simulink model "EngineModel_student2"  (R2016a)
settings: Solver=ode3  StartTime=0.0  StopTime=1*sim_time  FixedStep=stepsize  RelTol=1e-3
values from neighbouring files (symbols this model uses):
  AFR_effective = max(AFR_stoich,AFR)    [EM3.m]    (also in workspace.mat = 14.7)
  Bore = 73.4*10^-3    (= 0.0734)    [EM3.m]    (also in workspace.mat)
  Cd = 0.35    [EM3.m]    (also in workspace.mat)
  ConRod = 137.2*10^-3    (= 0.1372)    [EM3.m]    (also in workspace.mat)
  CrankRadius = Stroke/2    (= 0.0363)    [EM3.m]    (also in workspace.mat)
  engine_speed = 3000    [EM3.m]    (also in workspace.mat)
  gma = 1.32    [EM3.m]    (also in workspace.mat)
  LHV = 44400*10^3    (= 44400000)    [EM3.m]    (also in workspace.mat)
  m_0 = P_0*(V_comp)/(R*T_air)    (= 3.64160478062e-05)    [EM3.m]    (also in workspace.mat)
  MAP = 80000    [EM3.m]    (also in workspace.mat)
  Nr_of_valves = 2    [EM3.m]    (also in workspace.mat)
  P_0 = 100000    [EM3.m]    (also in workspace.mat)
  P_exhaust = 120000    [EM3.m]    (also in workspace.mat)
  R = 287    [EM3.m]    (also in workspace.mat)
  Rho = 1.27    [EM3.m]    (also in workspace.mat)
  T_air = 323    [EM3.m]    (also in workspace.mat)
  V_comp = V_cyl/(CR-1)    (= 3.37580404769e-05)    [EM3.m]    (also in workspace.mat)
  V_sonic = 20.0457*sqrt(T_air)    [EM3.m]    (also in workspace.mat = 360.265344687)
  Valve_dia = 30*10^-3    (= 0.03)    [EM3.m]    (also in workspace.mat)
  Valve_lift = 9*10^-3    (= 0.009)    [EM3.m]    (also in workspace.mat)
settings Model: Creator=htsauto  LastModifiedBy=Job
settings DataIOCC: LimitDataPoints=on  SaveFormat=Array  SignalLoggingSaveFormat=ModelDataLogs
settings OptimizationCC: ExpressionDepthLimit=2147483647
settings DebuggingCC: UnderspecifiedInitializationDetection=Classic  MergeDetectMultiDrivingBlocksExec=none  SolverPrmCheckMsg=warning  FcnCallInpInsideContextMsg=UseLocalSettings  StateNameClashWarn=warning
settings HardwareCC: ProdBitPerPointer=32  ProdLargestAtomicFloat=None  ProdIntDivRoundTo=Undefined  ProdEndianess=Unspecified  ProdWordSize=32  ProdHWDeviceType=32-bit Generic
settings ModelReferenceCC: PropagateSignalLabelsOutOfModel=off
settings GRTTargetCC: CombineOutputUpdateFcns=off  GRTInterface=on
settings ConfigComp: CovModelRefEnable=Off  CovSFcnEnable=off

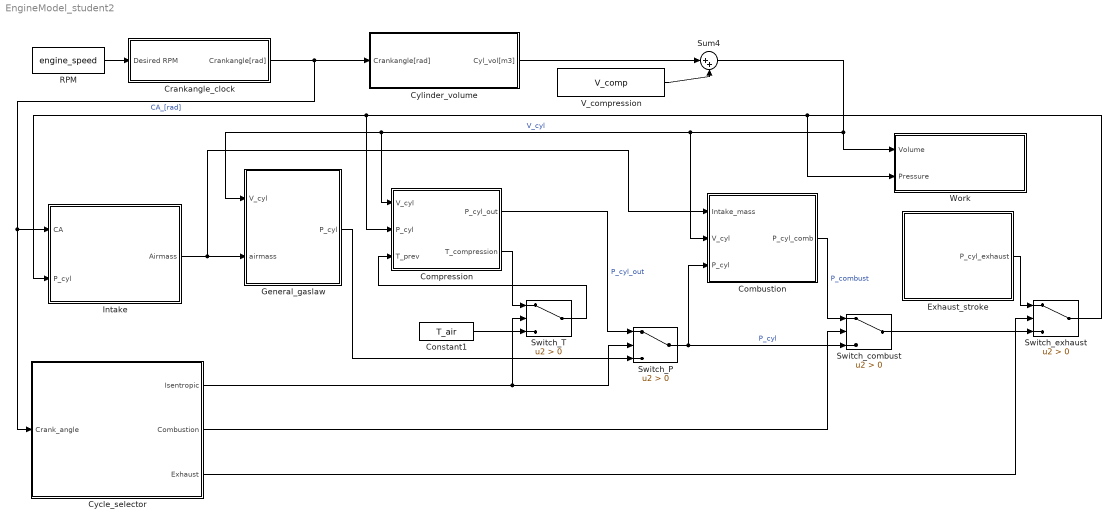
== system EngineModel_student2 ==
  Combustion : Subsystem
  Compression : Subsystem
  Constant1 : Constant  Value=T_air
  Crankangle_clock : Subsystem
  Cycle_selector : Subsystem
  Cylinder_volume : Subsystem
  Exhaust_stroke : Subsystem
  General_gaslaw : Subsystem
  Intake : Subsystem
  RPM : Constant  Value=engine_speed
  Sum4 : Sum  Inputs=|++
  Switch_P : Switch  Criteria=u2 > Threshold
  Switch_T : Switch  Criteria=u2 > Threshold
  Switch_combust : Switch  Criteria=u2 > Threshold
  Switch_exhaust : Switch  Criteria=u2 > Threshold
  V_compression : Constant  Value=V_comp
  Work : Subsystem
  wires:
  Sum4/1 -> Combustion/2(V_cyl), General_gaslaw/1(V_cyl), Compression/1(V_cyl), Work/1(Volume)  "V_cyl"
  RPM/1 -> Crankangle_clock/1(Desired RPM)
  Compression/1(P_cyl_out) -> Switch_P/1  "P_cyl_out"
  Compression/2(T_compression) -> Switch_T/1
  Switch_P/1 -> Switch_combust/3, Combustion/3(P_cyl)  "P_cyl"
  Combustion/1(P_cyl_comb) -> Switch_combust/1  "P_combust"
  Crankangle_clock/1(Crankangle[rad]) -> Cycle_selector/1(Crank_angle), Intake/1(CA), Cylinder_volume/1(Crankangle[rad])  "CA_[rad]"
  Switch_combust/1 -> Switch_exhaust/3
  Exhaust_stroke/1(P_cyl_exhaust) -> Switch_exhaust/1
  Cycle_selector/2(Combustion) -> Switch_combust/2
  Cycle_selector/3(Exhaust) -> Switch_exhaust/2
  Intake/1(Airmass) -> Combustion/1(Intake_mass), General_gaslaw/2(airmass)
  General_gaslaw/1(P_cyl) -> Switch_P/3
  Switch_exhaust/1 -> Work/2(Pressure), Intake/2(P_cyl), Compression/2(P_cyl)
  Switch_T/1 -> Compression/3(T_prev)
  Constant1/1 -> Switch_T/3
  Cycle_selector/1(Isentropic) -> Switch_P/2, Switch_T/2
  Cylinder_volume/1(Cyl_vol[m3]) -> Sum4/1
  V_compression/1 -> Sum4/2

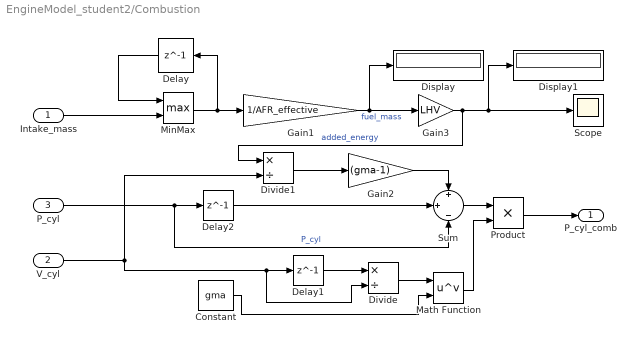
== system EngineModel_student2/Combustion ==
  Intake_mass : Inport
  V_cyl : Inport  Port=2
  P_cyl : Inport  Port=3
  Constant : Constant  Value=gma
  Delay : Delay  DelayLength=1  InitialCondition=0
  Delay1 : Delay  DelayLength=1
  Delay2 : Delay  DelayLength=1
  Display : Display
  Display1 : Display
  Divide : Product  Inputs=*/
  Divide1 : Product  Inputs=*/
  Gain1 : Gain  Gain=1/AFR_effective
  Gain2 : Gain  Gain=(gma-1)
  Gain3 : Gain  Gain=LHV
  Math Function : Math  Operator=pow  SaturateOnIntegerOverflow=on
  MinMax : MinMax  Function=max  Inputs=2
  Product : Product
  Scope : Scope
  Sum : Sum  Inputs=+|+|-
  P_cyl_comb : Outport
  wires:
  Intake_mass/1 -> MinMax/2
  MinMax/1 -> Delay/1, Gain1/1
  Gain1/1 -> Gain3/1, Display/1  "fuel_mass"
  Gain3/1 -> Scope/1, Display1/1, Divide1/1  "added_energy"
  Delay/1 -> MinMax/1
  Delay1/1 -> Divide/1
  Divide/1 -> Math Function/1
  Constant/1 -> Math Function/2
  Product/1 -> P_cyl_comb/1
  V_cyl/1 -> Divide1/2, Divide/2, Delay1/1
  P_cyl/1 -> Sum/3, Delay2/1  "P_cyl"
  Divide1/1 -> Gain2/1
  Sum/1 -> Product/1
  Gain2/1 -> Sum/1
  Delay2/1 -> Sum/2
  Math Function/1 -> Product/2

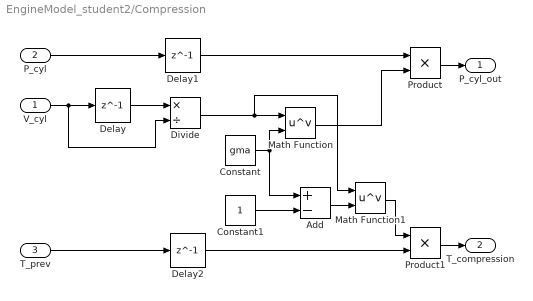
== system EngineModel_student2/Compression ==
  V_cyl : Inport
  P_cyl : Inport  Port=2
  T_prev : Inport  Port=3
  Add : Sum  Inputs=+-
  Constant : Constant  Value=gma
  Constant1 : Constant
  Delay : Delay  DelayLength=1  InitialCondition=0
  Delay1 : Delay  DelayLength=1
  Delay2 : Delay  DelayLength=1
  Divide : Product  Inputs=*/
  Math Function : Math  Operator=pow  SaturateOnIntegerOverflow=on
  Math Function1 : Math  Operator=pow  SaturateOnIntegerOverflow=on
  Product : Product
  Product1 : Product
  P_cyl_out : Outport
  T_compression : Outport  Port=2
  wires:
  V_cyl/1 -> Delay/1, Divide/2
  Math Function/1 -> Product/2
  Constant/1 -> Math Function/2, Add/1
  Constant1/1 -> Add/2
  Add/1 -> Math Function1/2
  Math Function1/1 -> Product1/1
  Product1/1 -> T_compression/1
  P_cyl/1 -> Delay1/1
  Divide/1 -> Math Function1/1, Math Function/1
  T_prev/1 -> Delay2/1
  Product/1 -> P_cyl_out/1
  Delay/1 -> Divide/1
  Delay1/1 -> Product/1
  Delay2/1 -> Product1/2

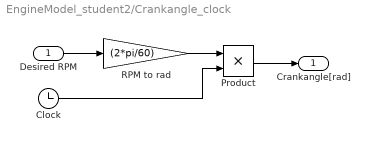
== system EngineModel_student2/Crankangle_clock ==
  Desired RPM : Inport
  Clock : Clock
  Product : Product
  RPM to rad : Gain  Gain=(2*pi/60)
  Crankangle[rad] : Outport
  wires:
  Desired RPM/1 -> RPM to rad/1
  RPM to rad/1 -> Product/1
  Clock/1 -> Product/2
  Product/1 -> Crankangle[rad]/1

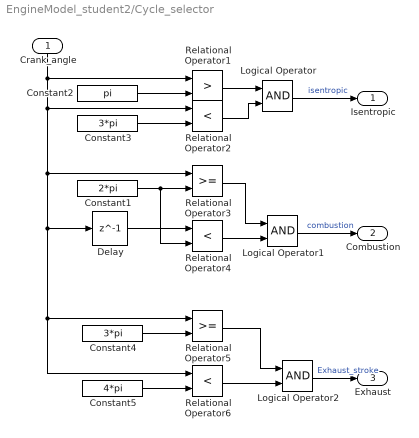
== system EngineModel_student2/Cycle_selector ==
  Crank_angle : Inport
  Constant1 : Constant  Value=2*pi
  Constant2 : Constant  Value=pi
  Constant3 : Constant  Value=3*pi
  Constant4 : Constant  Value=3*pi
  Constant5 : Constant  Value=4*pi
  Delay : Delay  DelayLength=1  InitialCondition=P_0
  Logical Operator : Logic  AllPortsSameDT=off  OutDataTypeStr=boolean
  Logical Operator1 : Logic  AllPortsSameDT=off  OutDataTypeStr=boolean
  Logical Operator2 : Logic  AllPortsSameDT=off  OutDataTypeStr=boolean
  Relational Operator1 : RelationalOperator  Operator=>  OutDataTypeStr=boolean
  Relational Operator2 : RelationalOperator  Operator=<  OutDataTypeStr=boolean
  Relational Operator3 : RelationalOperator  OutDataTypeStr=boolean
  Relational Operator4 : RelationalOperator  Operator=<  OutDataTypeStr=boolean
  Relational Operator5 : RelationalOperator  OutDataTypeStr=boolean
  Relational Operator6 : RelationalOperator  Operator=<  OutDataTypeStr=boolean
  Isentropic : Outport
  Combustion : Outport  Port=2
  Exhaust : Outport  Port=3
  wires:
  Relational Operator6/1 -> Logical Operator2/2
  Logical Operator2/1 -> Exhaust/1  "Exhaust_stroke"
  Relational Operator5/1 -> Logical Operator2/1
  Constant4/1 -> Relational Operator5/2
  Logical Operator/1 -> Isentropic/1  "isentropic"
  Relational Operator3/1 -> Logical Operator1/1
  Relational Operator4/1 -> Logical Operator1/2
  Logical Operator1/1 -> Combustion/1  "combustion"
  Constant2/1 -> Relational Operator1/2
  Constant1/1 -> Relational Operator4/2, Relational Operator3/2
  Relational Operator2/1 -> Logical Operator/2
  Relational Operator1/1 -> Logical Operator/1
  Delay/1 -> Relational Operator4/1
  Constant3/1 -> Relational Operator2/2
  Constant5/1 -> Relational Operator6/2
  Crank_angle/1 -> Relational Operator6/1, Relational Operator5/1, Delay/1, Relational Operator3/1, Relational Operator2/1, Relational Operator1/1

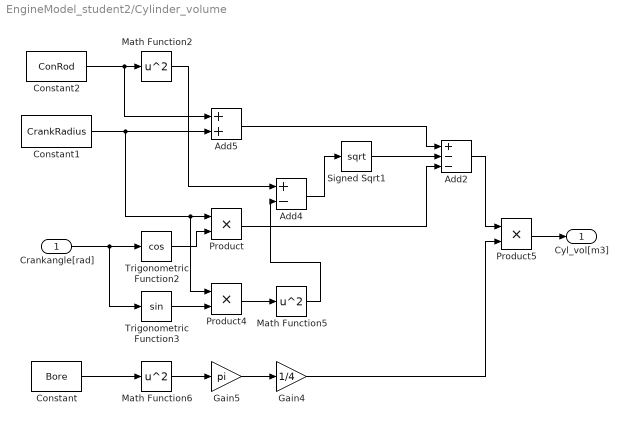
== system EngineModel_student2/Cylinder_volume ==
  Crankangle[rad] : Inport
  Add2 : Sum  Inputs=+--
  Add4 : Sum  Inputs=+-
  Add5 : Sum
  Constant : Constant  Value=Bore
  Constant1 : Constant  Value=CrankRadius
  Constant2 : Constant  Value=ConRod
  Gain4 : Gain  Gain=1/4
  Gain5 : Gain  Gain=pi
  Math Function2 : Math  Operator=square  SaturateOnIntegerOverflow=on
  Math Function5 : Math  Operator=square  SaturateOnIntegerOverflow=on
  Math Function6 : Math  Operator=square  SaturateOnIntegerOverflow=on
  Product : Product
  Product4 : Product
  Product5 : Product
  Signed Sqrt1 : Sqrt  SaturateOnIntegerOverflow=on
  Trigonometric Function2 : Trigonometry  Operator=cos
  Trigonometric Function3 : Trigonometry
  Cyl_vol[m3] : Outport
  wires:
  Constant1/1 -> Product4/1, Product/1, Add5/2
  Constant2/1 -> Math Function2/1, Add5/1
  Add5/1 -> Add2/1
  Trigonometric Function2/1 -> Product/2
  Math Function2/1 -> Add4/1
  Trigonometric Function3/1 -> Product4/2
  Product4/1 -> Math Function5/1
  Math Function5/1 -> Add4/2
  Add4/1 -> Signed Sqrt1/1
  Constant/1 -> Math Function6/1
  Signed Sqrt1/1 -> Add2/2
  Product/1 -> Add2/3
  Add2/1 -> Product5/1
  Product5/1 -> Cyl_vol[m3]/1
  Gain4/1 -> Product5/2
  Math Function6/1 -> Gain5/1
  Gain5/1 -> Gain4/1
  Crankangle[rad]/1 -> Trigonometric Function3/1, Trigonometric Function2/1

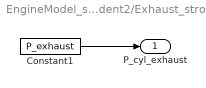
== system EngineModel_student2/Exhaust_stroke ==
  Constant1 : Constant  Value=P_exhaust
  P_cyl_exhaust : Outport
  wires:
  Constant1/1 -> P_cyl_exhaust/1

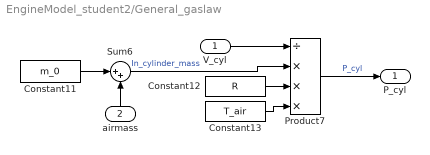
== system EngineModel_student2/General_gaslaw ==
  V_cyl : Inport
  airmass : Inport  Port=2
  Constant11 : Constant  Value=m_0
  Constant12 : Constant  Value=R
  Constant13 : Constant  Value=T_air
  Product7 : Product  Inputs=/***  RndMeth=Zero
  Sum6 : Sum  Inputs=|++
  P_cyl : Outport
  wires:
  Constant12/1 -> Product7/3
  Constant13/1 -> Product7/4
  Product7/1 -> P_cyl/1  "P_cyl"
  Sum6/1 -> Product7/2  "In_cylinder_mass"
  Constant11/1 -> Sum6/1
  airmass/1 -> Sum6/2
  V_cyl/1 -> Product7/1

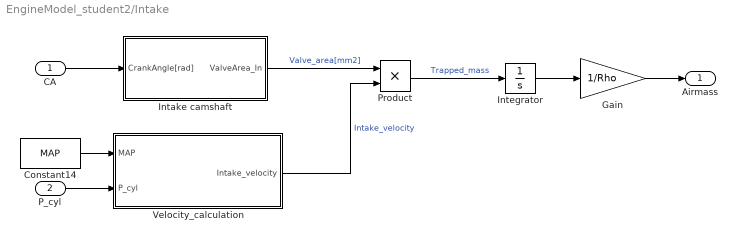
== system EngineModel_student2/Intake ==
  CA : Inport
  P_cyl : Inport  Port=2
  Constant14 : Constant  Value=MAP
  Gain : Gain  Gain=1/Rho
  Intake camshaft : Subsystem
  Integrator : Integrator
  Product : Product
  Velocity_calculation : Subsystem
  Airmass : Outport
  wires:
  Intake camshaft/1(ValveArea_In) -> Product/1  "Valve_area[mm2]"
  Velocity_calculation/1(Intake_velocity) -> Product/2  "Intake_velocity"
  Constant14/1 -> Velocity_calculation/1(MAP)
  CA/1 -> Intake camshaft/1(CrankAngle[rad])
  Product/1 -> Integrator/1  "Trapped_mass"
  Integrator/1 -> Gain/1
  Gain/1 -> Airmass/1
  P_cyl/1 -> Velocity_calculation/2(P_cyl)

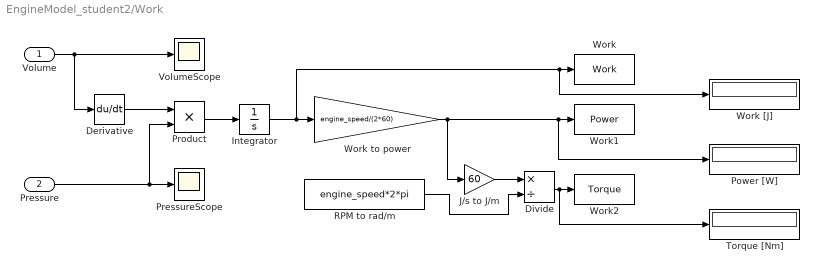
== system EngineModel_student2/Work ==
  Volume : Inport
  Pressure : Inport  Port=2
  Derivative : Derivative
  Divide : Product  Inputs=*/
  Integrator : Integrator
  J/s to J/m : Gain  Gain=60
  Power [W] : Display
  PressureScope : Scope
  Product : Product
  RPM to rad/m : Constant  Value=engine_speed*2*pi
  Torque [Nm] : Display
  VolumeScope : Scope
  Work : ToWorkspace  VariableName=Work  SampleTime=-1
      settings: MaxDataPoints=1
  Work [J] : Display
  Work to power : Gain  Gain=engine_speed/(2*60)
  Work1 : ToWorkspace  VariableName=Power  SampleTime=-1
      settings: MaxDataPoints=1
  Work2 : ToWorkspace  VariableName=Torque  SampleTime=-1
      settings: MaxDataPoints=1
  wires:
  Pressure/1 -> Product/2, PressureScope/1
  Integrator/1 -> Work [J]/1, Work/1, Work to power/1
  Volume/1 -> Derivative/1, VolumeScope/1
  Derivative/1 -> Product/1
  Product/1 -> Integrator/1
  Work to power/1 -> Power [W]/1, Work1/1, J/s to J/m/1
  J/s to J/m/1 -> Divide/1
  RPM to rad/m/1 -> Divide/2
  Divide/1 -> Torque [Nm]/1, Work2/1

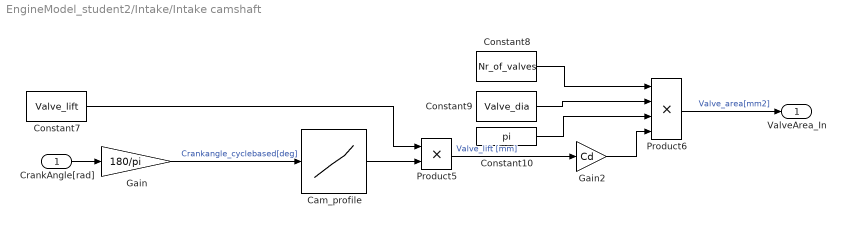
== system EngineModel_student2/Intake/Intake camshaft ==
  CrankAngle[rad] : Inport
  Cam_profile : Lookup_n-D  NumberOfTableDimensions=1  BreakpointsForDimension1=[0,10,20,30,40,50,60,70,80,90,100,110,120,130,140,150,160,170,180,190,200,210]  Table=[0,0.05,0.1,0.2,0.3,0.5,0.65,0.8,0.9,0.95,1,1,0.95,0.9,0.8,0.65,0.5,0.3,0.2,0.1,0.05,0]  ExtrapMethod=Clip  UseLastTableValue=on  RndMeth=Simplest  InputSameDT=on
  Constant10 : Constant  Value=pi
  Constant7 : Constant  Value=Valve_lift
  Constant8 : Constant  Value=Nr_of_valves
  Constant9 : Constant  Value=Valve_dia
  Gain : Gain  Gain=180/pi
  Gain2 : Gain  Gain=Cd
  Product5 : Product  RndMeth=Zero
  Product6 : Product  Inputs=4  RndMeth=Zero
  ValveArea_In : Outport
  wires:
  Cam_profile/1 -> Product5/2
  Product5/1 -> Gain2/1  "Valve_lift [mm]"
  Constant8/1 -> Product6/1
  Constant9/1 -> Product6/2
  Constant10/1 -> Product6/3
  Product6/1 -> ValveArea_In/1  "Valve_area[mm2]"
  CrankAngle[rad]/1 -> Gain/1
  Constant7/1 -> Product5/1
  Gain2/1 -> Product6/4
  Gain/1 -> Cam_profile/1  "Crankangle_cyclebased[deg]"

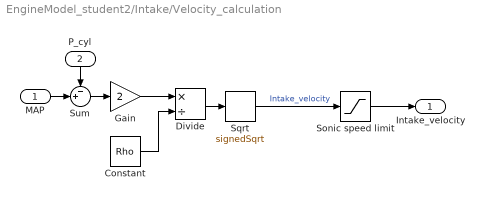
== system EngineModel_student2/Intake/Velocity_calculation ==
  MAP : Inport
  P_cyl : Inport  Port=2
  Constant : Constant  Value=Rho
  Divide : Product  Inputs=*/
  Gain : Gain  Gain=2
  Sonic speed limit : Saturate  UpperLimit=V_sonic  LowerLimit=-V_sonic
  Sqrt : Sqrt  Operator=signedSqrt  SaturateOnIntegerOverflow=on
  Sum : Sum  Inputs=-+|
  Intake_velocity : Outport
  wires:
  Sqrt/1 -> Sonic speed limit/1  "Intake_velocity"
  Sonic speed limit/1 -> Intake_velocity/1
  MAP/1 -> Sum/2
  P_cyl/1 -> Sum/1
  Sum/1 -> Gain/1
  Gain/1 -> Divide/1
  Constant/1 -> Divide/2
  Divide/1 -> Sqrt/1
